simulink model "sltestBasicCruiseControlBaseline"  (R2024a)
settings: Solver=FixedStepDiscrete  StartTime=0.0  StopTime=1  FixedStep=0.01  RelTol=1e-3  EnableMultiTasking=on
PostLoadFcn:
  | load('sltest_cruise_control_hierbus.mat');
undefined symbols (not defined in the file or in its folder): DiscIntNeverNeededParam
libraries: SignalEditorBlockLib x1
settings Model: Creator=The MathWorks, Inc.  LastModifiedBy=The MathWorks, Inc.
settings SolverCC: AlgebraicLoopSolver=TrustRegion
settings DataIOCC: LimitDataPoints=on  SaveFormat=Array  ReturnWorkspaceOutputs=off
settings OptimizationCC: ConditionallyExecuteInputs=off  DefaultParameterBehavior=Inlined  InlineInvariantSignals=on  ReuseModelBlockBuffer=off  ExpressionDepthLimit=2147483647  InitFltsAndDblsToZero=on  EfficientMapNaN2IntZero=off  LifeSpan=inf
settings DebuggingCC: SaveWithParameterizedLinksMsg=none  UnderspecifiedInitializationDetection=Classic  MergeDetectMultiDrivingBlocksExec=none  SignalResolutionControl=TryResolveAllWithWarning  SolverPrmCheckMsg=warning  FcnCallInpInsideContextMsg=warning  UnconnectedInputMsg=warning  UnconnectedOutputMsg=warning  UnconnectedLineMsg=warning  AllowSymbolicDim=off  StateNameClashWarn=warning  SFUnexpectedBacktrackingDiag=warning  SFNoUnconditionalDefaultTransitionDiag=warning  SFExecutionAtInitializationDiag=none  ArithmeticOperatorsInVariantConditions=warning
settings HardwareCC: ProdBitPerPointer=32  ProdBitPerSizeT=32  ProdBitPerPtrDiffT=32  ProdLargestAtomicFloat=None  ProdIntDivRoundTo=Undefined  ProdEndianess=Unspecified  ProdWordSize=32  ProdHWDeviceType=32-bit Generic
settings ModelReferenceCC: EnableRefExpFcnMdlSchedulingChecks=on  PropagateSignalLabelsOutOfModel=off
settings SFSimCC: SimUseLocalCustomCode=off  CustomCodeUndefinedFunction=UseInterfaceOnly
settings RTWCC: RTWUseLocalCustomCode=off  GPUComputeCapability=3.5  DLArmComputeVersion=19.05
settings CodeAppCC: StateflowObjectComments=on
settings GRTTargetCC: TargetFcnLib=ansi_tfl_tmw.mat  TargetLangStandard=C89/C90 (ANSI)  CombineOutputUpdateFcns=off  GRTInterface=on
settings ConfigComp: CovMetricSettings=dcmse  DVMaxProcessTime=60  DVMakeOutputFilesUnique=off  DVParameterConfiguration=UseParameterConfigFile  DVParameters=on  DVModelCoverageObjectives=MCDC  DVMaxTestCaseSteps=500  DVTestSuiteOptimization=CombinedObjectives  DVAssertions=EnableAll  DVProofAssumptions=EnableAll  DVDetectActiveLogic=on  DVProvingStrategy=FindViolation

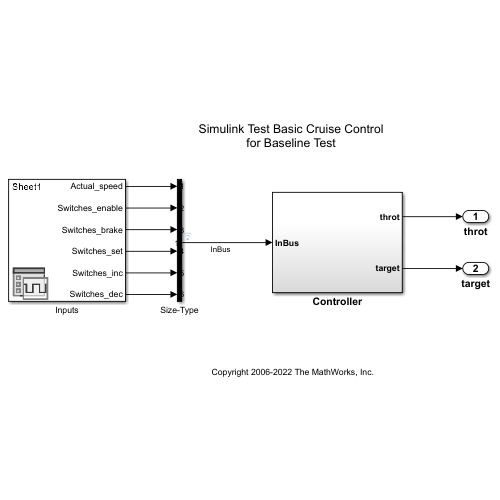
[thumbnail: Simulink's stored preview of the top-level diagram]
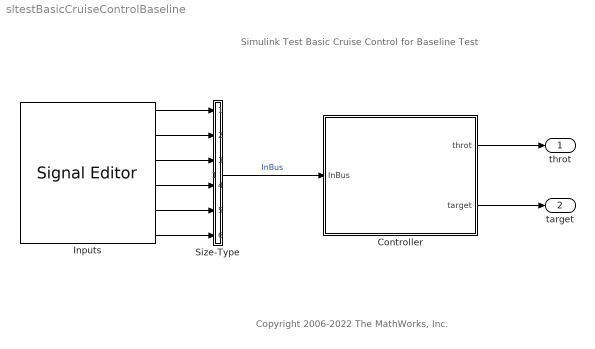
== system sltestBasicCruiseControlBaseline ==
  note: Simulink Test Basic Cruise Control
      | for Baseline Test
  note: Copyright 2006-2022 The MathWorks, Inc.
  Controller : Subsystem
  Inputs : SignalEditorBlockLib/Signal Editor  FileName=dataset_sltestBasicCruise.mat  ActiveScenario=Sheet1  ActiveSignal=Switches_dec  IsBus=off  OutputBusObjectStr=Bus: BusObject  SampleTime=0  ZeroCross=off  OutputAfterFinalValue=Extrapolation  Unit=inherit  PreserveSignalName=on  ApplySigPropsToAllScenarios=on  ApplySigPropsToAllSignals=off
  Size-Type : Subsystem
  throt : Outport  VectorParamsAs1DForOutWhenUnconnected=off
  target : Outport  Port=2  VectorParamsAs1DForOutWhenUnconnected=off
  wires:
  Controller/2(target) -> target/1
  Inputs/1 -> Size-Type/1(In1)
  Inputs/2 -> Size-Type/2(In2)
  Inputs/3 -> Size-Type/3(In3)
  Inputs/4 -> Size-Type/4(In4)
  Inputs/5 -> Size-Type/5(In5)
  Inputs/6 -> Size-Type/6(In6)
  Controller/1(throt) -> throt/1
  Size-Type/1(Out1) -> Controller/1(InBus)  "InBus"

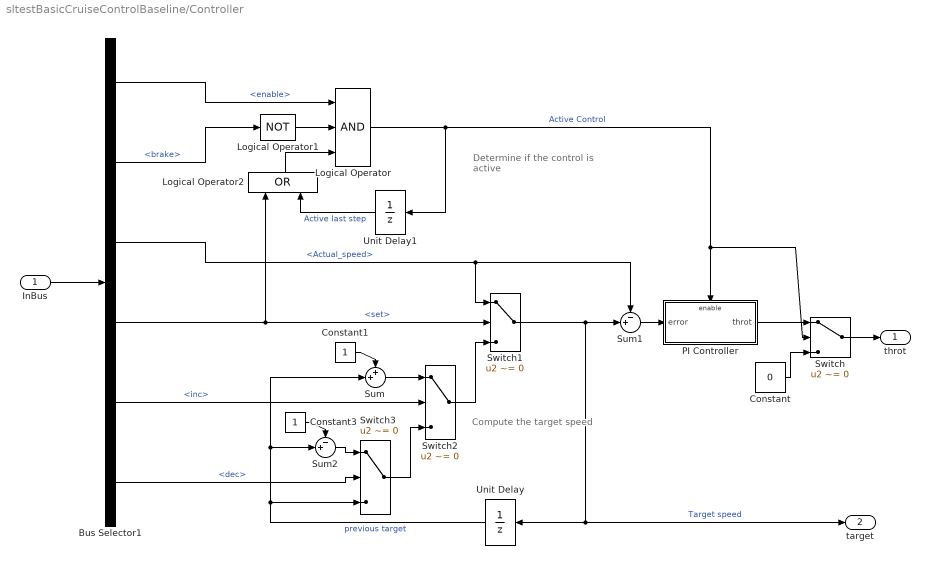
== system sltestBasicCruiseControlBaseline/Controller ==
  note: Determine if the
      | control is active
  note: Compute the
      | target speed
  InBus : Inport  OutDataTypeStr=Bus: InputBus
  Bus Selector1 : BusSelector  OutputSignals=Switches.enable,Switches.brake,Actual_speed,Switches.set,Switches.setIncDec.inc,Switches.setIncDec.dec
  Constant : Constant  Value=0
  Constant1 : Constant
  Constant3 : Constant
  Logical Operator : Logic  Inputs=3  AllPortsSameDT=off  OutDataTypeStr=boolean
  Logical Operator1 : Logic  Operator=NOT  AllPortsSameDT=off  OutDataTypeStr=boolean
  Logical Operator2 : Logic  Operator=OR  AllPortsSameDT=off  OutDataTypeStr=boolean
  PI Controller : Subsystem
  Sum : Sum  Inputs=++|
  Sum1 : Sum  Inputs=-+|
  Sum2 : Sum  Inputs=-+|
  Switch{,1..3} (4 alike) : Switch  Criteria=u2 ~= 0  SaturateOnIntegerOverflow=off  InputSameDT=off
  Unit Delay : UnitDelay  SampleTime=0.01  HasFrameUpgradeWarning=on
  Unit Delay1 : UnitDelay  SampleTime=0.01  HasFrameUpgradeWarning=on
  throt : Outport  VectorParamsAs1DForOutWhenUnconnected=off
  target : Outport  Port=2  VectorParamsAs1DForOutWhenUnconnected=off
  wires:
  Sum/1 -> Switch2/1
  Switch3/1 -> Switch2/3
  Logical Operator/1 -> Unit Delay1/1, PI Controller/Enable, Switch/2  "Active Control"
  Sum1/1 -> PI Controller/1(error)
  InBus/1 -> Bus Selector1/1
  Bus Selector1/2 -> Logical Operator1/1  "<brake>"
  Constant1/1 -> Sum/1
  Bus Selector1/4 -> Logical Operator2/1, Switch1/2  "<set>"
  Switch2/1 -> Switch1/3
  Bus Selector1/3 -> Switch1/1, Sum1/1  "<Actual_speed>"
  Bus Selector1/1 -> Logical Operator/1  "<enable>"
  Switch/1 -> throt/1
  Bus Selector1/6 -> Switch3/2  "<dec>"
  Constant/1 -> Switch/3
  Unit Delay1/1 -> Logical Operator2/2  "Active last step"
  Switch1/1 -> Unit Delay/1, target/1, Sum1/2  "Target speed"
  Bus Selector1/5 -> Switch2/2  "<inc>"
  Logical Operator1/1 -> Logical Operator/2
  Sum2/1 -> Switch3/1
  Logical Operator2/1 -> Logical Operator/3
  PI Controller/1(throt) -> Switch/1
  Unit Delay/1 -> Sum/2, Sum2/2, Switch3/3  "previous target"
  Constant3/1 -> Sum2/1

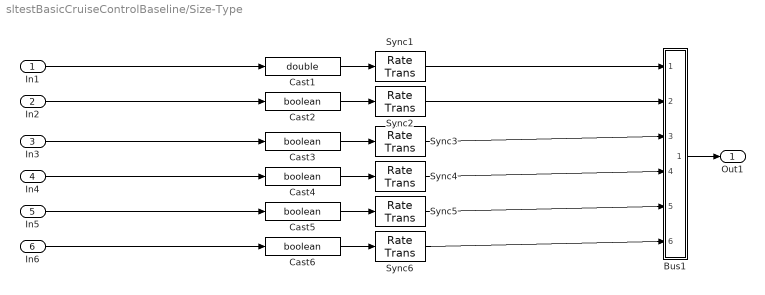
== system sltestBasicCruiseControlBaseline/Size-Type ==
  In1 : Inport
  In2 : Inport  Port=2
  In3 : Inport  Port=3
  In4 : Inport  Port=4
  In5 : Inport  Port=5
  In6 : Inport  Port=6
  Bus1 : Subsystem
  Cast1 : DataTypeConversion  OutDataTypeStr=double  RndMeth=Nearest
  Cast{2..6} (5 alike) : DataTypeConversion  OutDataTypeStr=boolean  RndMeth=Nearest
  Sync{1..6} (6 alike) : RateTransition  OutPortSampleTime=[0.01,0]
  Out1 : Outport  VectorParamsAs1DForOutWhenUnconnected=off
  wires:
  In1/1 -> Cast1/1
  Cast1/1 -> Sync1/1
  In2/1 -> Cast2/1
  Cast2/1 -> Sync2/1
  In3/1 -> Cast3/1
  Cast3/1 -> Sync3/1
  In4/1 -> Cast4/1
  Cast4/1 -> Sync4/1
  In5/1 -> Cast5/1
  Cast5/1 -> Sync5/1
  In6/1 -> Cast6/1
  Cast6/1 -> Sync6/1
  Sync1/1 -> Bus1/1(InputData(1).Actual_speed)
  Sync2/1 -> Bus1/2(InputData(1).Switches(1).enable)
  Sync3/1 -> Bus1/3(InputData(1).Switches(1).brake)
  Sync4/1 -> Bus1/4(InputData(1).Switches(1).set)
  Sync5/1 -> Bus1/5(InputData(1).Switches(1).setIncDec(1).inc)
  Sync6/1 -> Bus1/6(InputData(1).Switches(1).setIncDec(1).dec)
  Bus1/1(Out) -> Out1/1

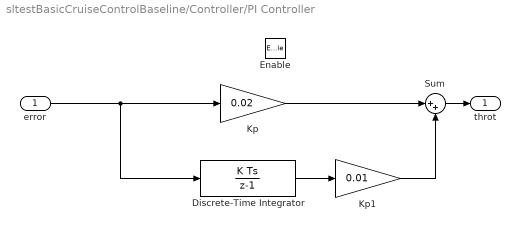
== system sltestBasicCruiseControlBaseline/Controller/PI Controller ==
  error : Inport
  Enable : EnablePort  PropagateVarSize=During execution
  Discrete-Time Integrator : DiscreteIntegrator  SampleTime=0.01  LimitOutput=on  UpperSaturationLimit=5  LowerSaturationLimit=-5  ICPrevOutput=DiscIntNeverNeededParam  ICPrevScaledInput=DiscIntNeverNeededParam
  Kp : Gain  Gain=0.02
  Kp1 : Gain  Gain=0.01
  Sum : Sum  Inputs=|++
  throt : Outport  InitialOutput=0  VectorParamsAs1DForOutWhenUnconnected=off
  wires:
  Kp/1 -> Sum/1
  Kp1/1 -> Sum/2
  Discrete-Time Integrator/1 -> Kp1/1
  error/1 -> Kp/1, Discrete-Time Integrator/1
  Sum/1 -> throt/1

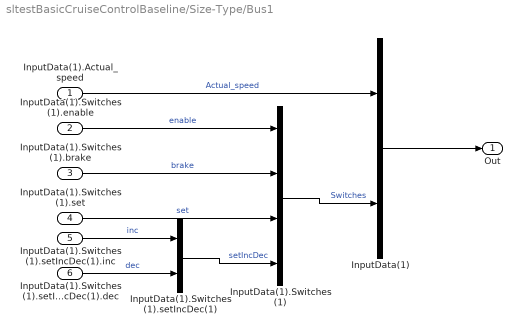
== system sltestBasicCruiseControlBaseline/Size-Type/Bus1 ==
  InputData(1).Actual_speed : Inport
  InputData(1).Switches(1).enable : Inport  Port=2
  InputData(1).Switches(1).brake : Inport  Port=3
  InputData(1).Switches(1).set : Inport  Port=4
  InputData(1).Switches(1).setIncDec(1).inc : Inport  Port=5
  InputData(1).Switches(1).setIncDec(1).dec : Inport  Port=6
  InputData(1) : BusCreator  Inputs=2  OutDataTypeStr=Bus: InputBus  NonVirtualBus=on
  InputData(1).Switches(1) : BusCreator  Inputs=4  OutDataTypeStr=Bus: Switches  NonVirtualBus=on
  InputData(1).Switches(1).setIncDec(1) : BusCreator  Inputs=2  OutDataTypeStr=Bus: setpoint  NonVirtualBus=on
  Out : Outport  VectorParamsAs1DForOutWhenUnconnected=off
  wires:
  InputData(1).Switches(1).setIncDec(1).inc/1 -> InputData(1).Switches(1).setIncDec(1)/1  "inc"
  InputData(1).Switches(1).setIncDec(1).dec/1 -> InputData(1).Switches(1).setIncDec(1)/2  "dec"
  InputData(1).Switches(1).enable/1 -> InputData(1).Switches(1)/1  "enable"
  InputData(1).Switches(1).brake/1 -> InputData(1).Switches(1)/2  "brake"
  InputData(1).Switches(1).set/1 -> InputData(1).Switches(1)/3  "set"
  InputData(1).Switches(1).setIncDec(1)/1 -> InputData(1).Switches(1)/4  "setIncDec"
  InputData(1).Actual_speed/1 -> InputData(1)/1  "Actual_speed"
  InputData(1).Switches(1)/1 -> InputData(1)/2  "Switches"
  InputData(1)/1 -> Out/1
